simulink model "solar_radiation_pressure"  (R2023a)
settings: Solver=VariableStepAuto  StartTime=0.0  StopTime=10.0  RelTol=1e-3
undefined symbols (not defined in the file or in its folder): km, m, s
libraries: aerolibconvert2 x2
settings Model: Creator=orous  LastModifiedBy=orous

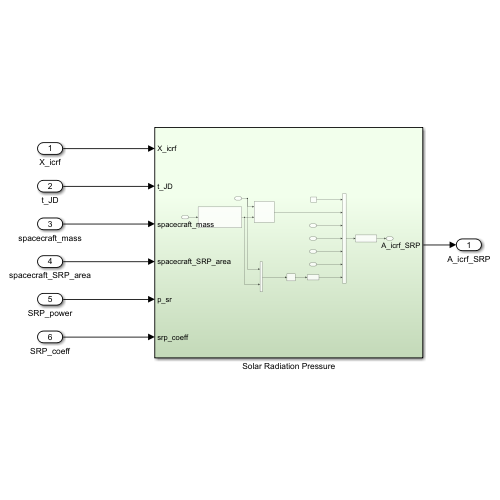
[thumbnail: Simulink's stored preview of the top-level diagram]
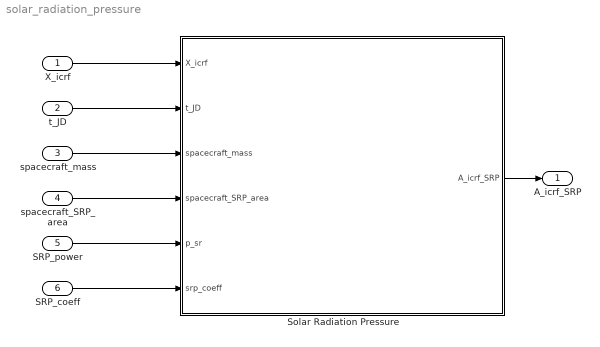
== system solar_radiation_pressure ==
  X_icrf : Inport
  t_JD : Inport  Port=2
  spacecraft_mass : Inport  Port=3
  spacecraft_SRP_area : Inport  Port=4
  SRP_power : Inport  Port=5
  SRP_coeff : Inport  Port=6
  Solar Radiation Pressure : Subsystem
  A_icrf_SRP : Outport
  wires:
  X_icrf/1 -> Solar Radiation Pressure/1(X_icrf)
  spacecraft_SRP_area/1 -> Solar Radiation Pressure/4(spacecraft_SRP_area)
  spacecraft_mass/1 -> Solar Radiation Pressure/3(spacecraft_mass)
  t_JD/1 -> Solar Radiation Pressure/2(t_JD)
  SRP_power/1 -> Solar Radiation Pressure/5(p_sr)
  SRP_coeff/1 -> Solar Radiation Pressure/6(srp_coeff)
  Solar Radiation Pressure/1(A_icrf_SRP) -> A_icrf_SRP/1

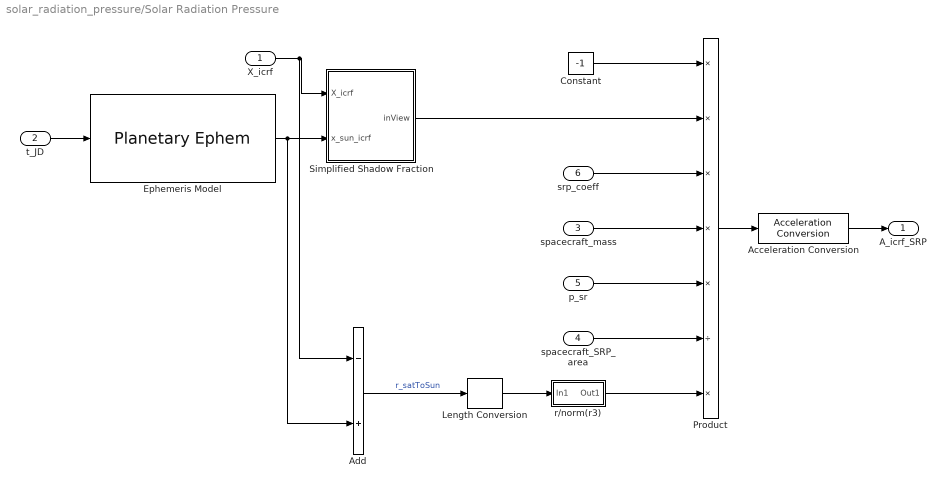
== system solar_radiation_pressure/Solar Radiation Pressure ==
  X_icrf : Inport
  t_JD : Inport  Port=2
  spacecraft_mass : Inport  Port=3
  spacecraft_SRP_area : Inport  Port=4
  p_sr : Inport  Port=5
  srp_coeff : Inport  Port=6
  Acceleration Conversion : aerolibconvert2/Acceleration Conversion  IU=m/s^2  OU=km/s^2
  Add : Sum  Inputs=-+
  Constant : Constant  Value=-1
  Ephemeris Model : PlanetaryEphem  target=Sun  outputVelocity=off
      settings: AttributesFormatString=|
      | %<nCenter> to %<nTarget>
      | JPL Model: %<de>
  Length Conversion : aerolibconvert2/Length Conversion  IU=km  OU=m
  Product : Product  Inputs=*****/*
  Simplified Shadow Fraction : Subsystem
  r/norm(r3) : Subsystem
  A_icrf_SRP : Outport
  wires:
  srp_coeff/1 -> Product/3
  Constant/1 -> Product/1
  Length Conversion/1 -> r/norm(r3)/1(In1)
  Ephemeris Model/1 -> Simplified Shadow Fraction/2(x_sun_icrf), Add/2
  t_JD/1 -> Ephemeris Model/1
  Add/1 -> Length Conversion/1  "r_satToSun"
  Simplified Shadow Fraction/1(inView) -> Product/2
  X_icrf/1 -> Simplified Shadow Fraction/1(X_icrf), Add/1
  spacecraft_mass/1 -> Product/4
  p_sr/1 -> Product/5
  spacecraft_SRP_area/1 -> Product/6
  r/norm(r3)/1(Out1) -> Product/7
  Product/1 -> Acceleration Conversion/1
  Acceleration Conversion/1 -> A_icrf_SRP/1

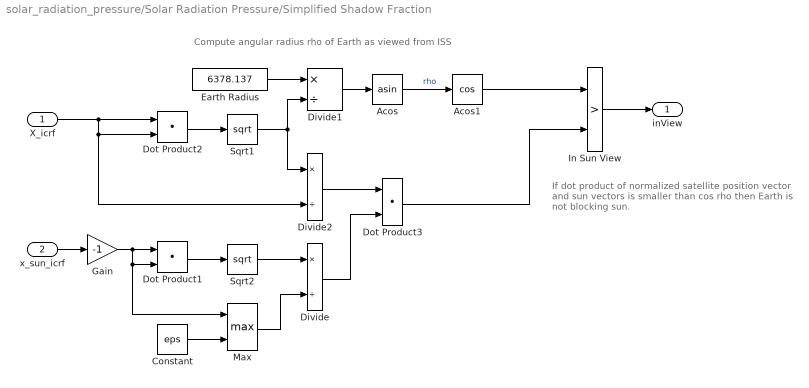
== system solar_radiation_pressure/Solar Radiation Pressure/Simplified Shadow Fraction ==
  note: Compute angular radius rho of Earth as viewed from ISS
  note: If dot product of normalized satellite position vector and sun vectors is smaller than cos rho then Earth is not blocking sun.
  X_icrf : Inport
  x_sun_icrf : Inport  Port=2  SampleTime=0
  Acos : Trigonometry  Operator=asin
  Acos1 : Trigonometry  Operator=cos
  Constant : Constant  Value=eps
  Divide : Product  Inputs=*/
  Divide1 : Product  Inputs=*/
  Divide2 : Product  Inputs=*/
  Dot Product1 : DotProduct  OutDataTypeStr=Inherit: Inherit via internal rule
  Dot Product2 : DotProduct  OutDataTypeStr=Inherit: Inherit via internal rule
  Dot Product3 : DotProduct  OutDataTypeStr=Inherit: Inherit via internal rule
  Earth Radius : Constant  Value=6378.137  VectorParams1D=off  SampleTime=0
  Gain : Gain  Gain=-1
  In Sun View : RelationalOperator  Operator=>  OutDataTypeStr=boolean  ZeroCross=off  RndMeth=Simplest  InputSameDT=off
  Max : MinMax  Function=max  Inputs=2
  Sqrt1 : Sqrt
  Sqrt2 : Sqrt
  inView : Outport  SampleTime=0
  wires:
  Gain/1 -> Max/1, Dot Product1/2, Dot Product1/1
  In Sun View/1 -> inView/1
  X_icrf/1 -> Divide2/2, Dot Product2/2, Dot Product2/1
  Earth Radius/1 -> Divide1/1
  Dot Product2/1 -> Sqrt1/1
  x_sun_icrf/1 -> Gain/1
  Sqrt1/1 -> Divide2/1, Divide1/2
  Divide1/1 -> Acos/1
  Acos/1 -> Acos1/1  "rho"
  Divide/1 -> Dot Product3/2
  Acos1/1 -> In Sun View/1
  Divide2/1 -> Dot Product3/1
  Dot Product3/1 -> In Sun View/2
  Sqrt2/1 -> Divide/1
  Dot Product1/1 -> Sqrt2/1
  Constant/1 -> Max/2
  Max/1 -> Divide/2

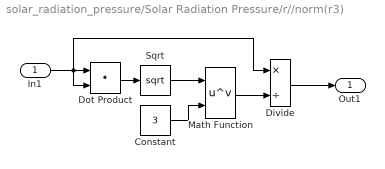
== system solar_radiation_pressure/Solar Radiation Pressure/r//norm(r3) ==
  In1 : Inport
  Constant : Constant  Value=3
  Divide : Product  Inputs=*/
  Dot Product : DotProduct  OutDataTypeStr=Inherit: Inherit via internal rule
  Math Function : Math  Operator=pow
  Sqrt : Sqrt
  Out1 : Outport
  wires:
  Math Function/1 -> Divide/2
  Constant/1 -> Math Function/2
  In1/1 -> Divide/1, Dot Product/2, Dot Product/1
  Sqrt/1 -> Math Function/1
  Dot Product/1 -> Sqrt/1
  Divide/1 -> Out1/1
